simulink model "check_Pressure_Drop_staticHeight"  (R2013b)
settings: Solver=ode45  StartTime=0.0  StopTime=10.0  RelTol=1e-3
libraries: carnot x2
settings Model: Creator=drhf  LastModifiedBy=drhf
settings DataIOCC: SignalLoggingSaveFormat=ModelDataLogs
settings OptimizationCC: ExpressionDepthLimit=2147483647
settings DebuggingCC: FcnCallInpInsideContextMsg=UseLocalSettings  StateNameClashWarn=warning
settings GRTTargetCC: CombineOutputUpdateFcns=off  GRTInterface=on

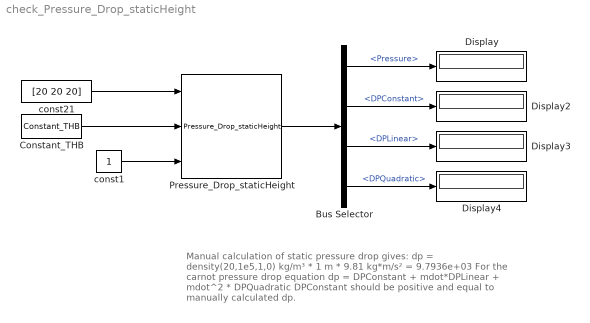
== system check_Pressure_Drop_staticHeight ==
  note: Manual calculation of static pressure drop gives:
      | dp = density(20,1e5,1,0) kg/m³ * 1 m  * 9.81 kg*m/s² = 9.7936e+03
      |
      | For the carnot pressure drop equation
      | dp = DPConstant + mdot*DPLinear + mdot^2 * DPQuadratic
      | DPConstant should be positive and equal to manually calculated dp.
  Bus Selector : BusSelector  OutputSignals=Pressure,DPConstant,DPLinear,DPQuadratic
  Constant_THB : carnot/Source/Simple/Constant_THB  t=40  mdot=100/3600  p=1e5  mID=Full Pressure Drop with Static Height  fluid=Water  mix=0  mix2=0  mix3=0  dia=1  hgt=0
  Display{,2..4} (4 alike) : Display
  Pressure_Drop_staticHeight : carnot/Basic/Pressure_Drop/Pressure_Drop_staticHeight
  const1 : Constant
  const21 : Constant  Value=[20 20 20]
  wires:
  Constant_THB/1 -> Pressure_Drop_staticHeight/2
  Pressure_Drop_staticHeight/1 -> Bus Selector/1
  Bus Selector/1 -> Display/1  "<Pressure>"
  Bus Selector/2 -> Display2/1  "<DPConstant>"
  Bus Selector/3 -> Display3/1  "<DPLinear>"
  Bus Selector/4 -> Display4/1  "<DPQuadratic>"
  const21/1 -> Pressure_Drop_staticHeight/1
  const1/1 -> Pressure_Drop_staticHeight/3
